simulink library "Dampers_Axle1_Interconnected"  (R2026a)
settings: Solver=VariableStepAuto
libraries: Damper_Basics x1
Description:
  | Component of Simscape Vehicle Templates Library
  | 
  | Copyright 2018-2026 The MathWorks, Inc.
settings Model: Creator=smiller  LastModifiedBy=smiller

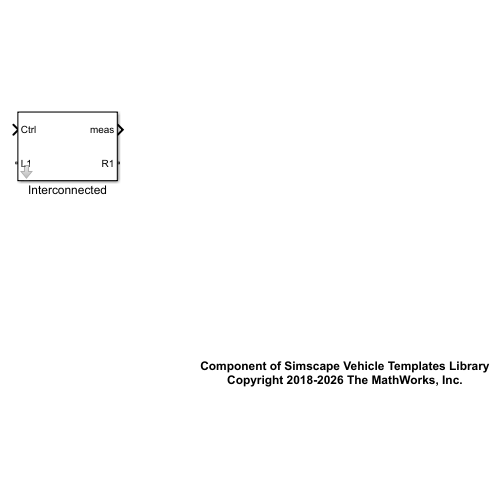
[thumbnail: Simulink's stored preview of the top-level diagram]
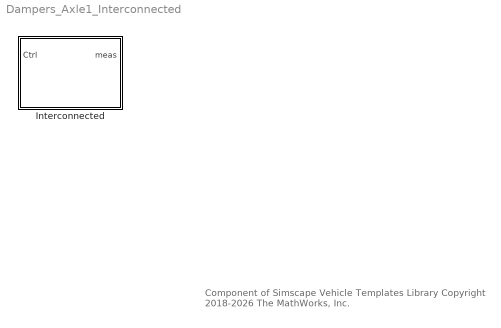
== system Dampers_Axle1_Interconnected ==
  note: Component of Simscape Vehicle Templates Library
      | Copyright 2018-2026 The MathWorks, Inc.
  Interconnected : Subsystem  VariantControl=Interconnected  mask(Interconnected Dampers){InitTriggerDropdown=0}
      mask prompts: InitTriggerDropdown "Initialization Trigger Dropdown"
      mask help: Dampers connected across an axle.
      mask init:
      | curblk = gcb;
      | 
      | % Trigger Mask Initialization for 
      | % variant subsystems below this level
      | sm_car_lib_maskInitTrigger(curblk);
      mask TypeOptions InitTriggerDropdown: 0 | 1

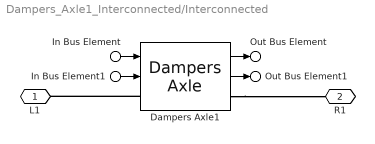
== system Dampers_Axle1_Interconnected/Interconnected ==
  In Bus Element1 : Inport  PortName=Ctrl  Element=R1
  In Bus Element : Inport  PortName=Ctrl  Element=L1
  Dampers Axle1 : Damper_Basics/Dampers Axle  VariantControl=Variant1  LabelModeActiveChoice=Linear  Damper=Damper.Axle1  VariantLabel=Damper.Axle1.class.Value  InitTriggerDropdown=0
      settings: AttributesFormatString=%<ActiveVariant>
  L1 : PMIOPort  Side=Left
  R1 : PMIOPort  Port=2  Side=Right
  Out Bus Element : Outport  VectorParamsAs1DForOutWhenUnconnected=off  PortName=meas  Element=L1
  Out Bus Element1 : Outport  VectorParamsAs1DForOutWhenUnconnected=off  PortName=meas  Element=R1
  wires:
  In Bus Element/1 -> Dampers Axle1/1
  In Bus Element1/1 -> Dampers Axle1/2
  Dampers Axle1/1 -> Out Bus Element/1
  Dampers Axle1/2 -> Out Bus Element1/1
  connections:
  Dampers Axle1/LConn1 -- L1/RConn1
  Dampers Axle1/RConn1 -- R1/RConn1
